simulink model "vJaco"  (R2014b)
settings: Solver=ode45  StartTime=0.0  StopTime=10  RelTol=1e-3
undefined symbols (not defined in the file or in its folder): JacFt
libraries: simulink x3
settings Model: Creator=Kelly  LastModifiedBy=heredia

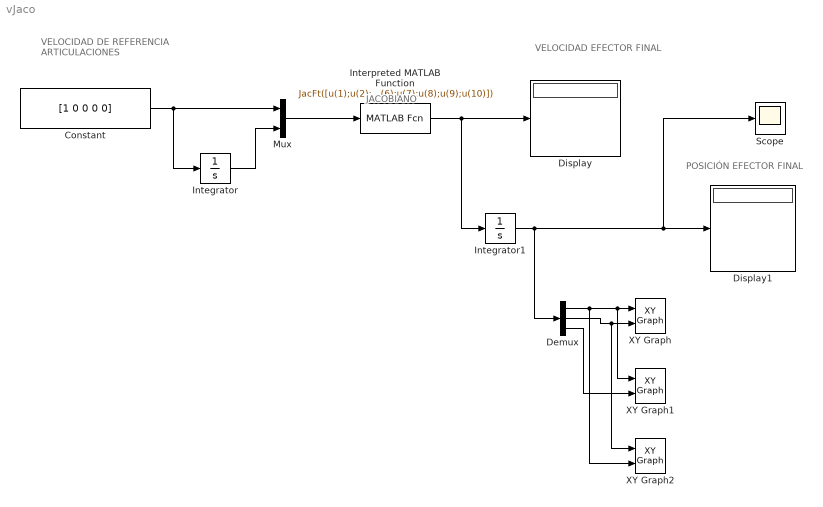
== system vJaco ==
  note: POSICIÓN EFECTOR FINAL
  note: VELOCIDAD
      | EFECTOR FINAL
  note: VELOCIDAD DE
      | REFERENCIA
      | ARTICULACIONES
  note: JACOBIANO
  Constant : Constant  Value=[1 0 0 0 0]
  Demux : Demux  Outputs=3
  Display : Display
  Display1 : Display
  Integrator : Integrator  InitialCondition=[0 pi/4 0 0 0]
  Integrator1 : Integrator  InitialCondition=[0.59 0 0.4]
  Interpreted MATLAB Function : MATLABFcn  MATLABFcn=JacFt([u(1);u(2);u(3);u(4);u(5)],[u(6);u(7);u(8);u(9);u(10)])
  Mux : Mux  Inputs=2
  Scope : Scope
  XY Graph : simulink/Sinks/XY Graph  xmin=-10  xmax=10  ymin=-10  ymax=10  st=-1
  XY Graph1 : simulink/Sinks/XY Graph  xmin=-10  xmax=10  ymin=-10  ymax=10  st=-1
  XY Graph2 : simulink/Sinks/XY Graph  xmin=-10  xmax=10  ymin=-10  ymax=10  st=-1
  wires:
  Constant/1 -> Integrator/1, Mux/1
  Integrator/1 -> Mux/2
  Mux/1 -> Interpreted MATLAB Function/1
  Interpreted MATLAB Function/1 -> Integrator1/1, Display/1
  Integrator1/1 -> Demux/1, Scope/1, Display1/1
  Demux/1 -> XY Graph2/2, XY Graph1/1, XY Graph/1
  Demux/2 -> XY Graph2/1, XY Graph/2
  Demux/3 -> XY Graph1/2
